simulink subsystem "brakePressure"  (R2023b)
settings: Solver=VariableStepAuto  StartTime=0.0  StopTime=10.0  RelTol=1e-3
libraries: brake_lib x4, Raptor_lib x4
settings Model: Creator=serga  LastModifiedBy=serga
settings OptimizationCC: ReuseModelBlockBuffer=off

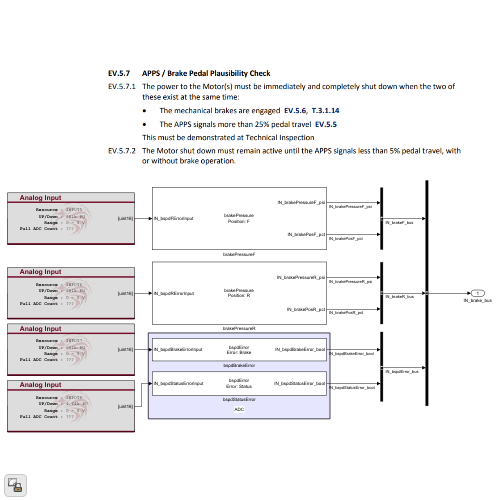
[thumbnail: Simulink's stored preview of the top-level diagram]
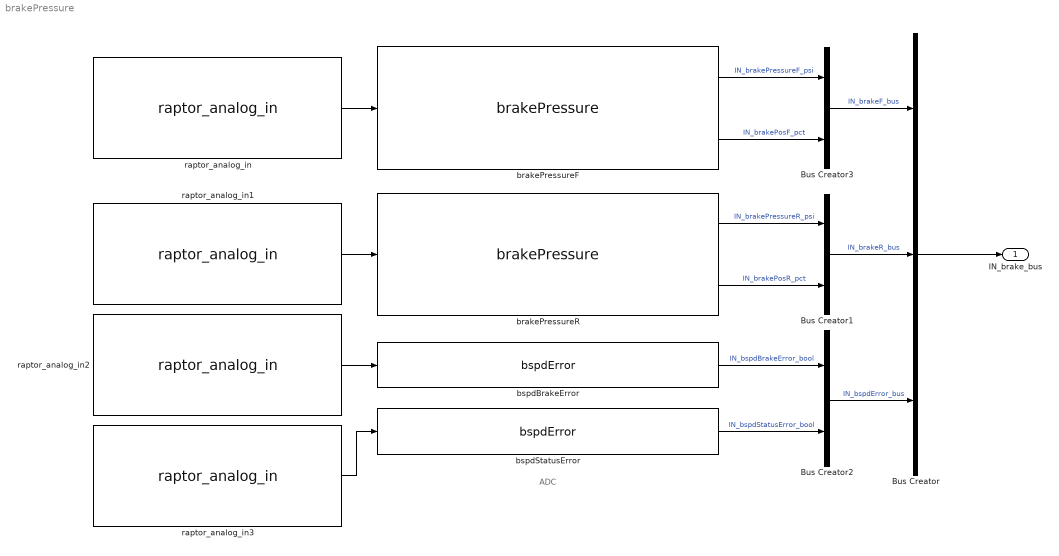
== system brakePressure ==
  note: ADC
  Bus Creator : BusCreator  Inputs=3
  Bus Creator1 : BusCreator  Inputs=2
  Bus Creator2 : BusCreator  Inputs=2
  Bus Creator3 : BusCreator  Inputs=2
  brakePressureF : brake_lib/brakePressure  pos='F'
  brakePressureR : brake_lib/brakePressure  pos='R'
  bspdBrakeError : brake_lib/bspdError  pos='Brake'
  bspdStatusError : brake_lib/bspdError  pos='Status'
  raptor_analog_in : Raptor_lib/Input & Output/raptor_analog_in  resourceValues=INPUT2|INPUT3|INPUT4|INPUT5|INPUT6|INPUT7|INPUT8|INPUT9|INPUT10|INPUT11|INPUT12|INPUT13|INPUT14|INPUT15|INPUT16|INPUT17|INPUT18|INPUT19|INPUT20|INPUT21|INPUT22|INPUT23|INPUT24|INPUT25|INPUT26|INPUT27|INPUT28|INPUT29|INPUT30|INPUT31|INPUT32|(None)  resource=INPUT4  rangeValues=0 - 5 V  range=0 - 5 V  filterrateValues=[]  filterrate='RAPTOR MASK DEFAULT'  resolutionValues=[]  resolution=[]  pullUDValues=422k PD  pullUD=422k PD
      settings: SourceProductName=Raptor
  raptor_analog_in1 : Raptor_lib/Input & Output/raptor_analog_in  resourceValues=INPUT2|INPUT3|INPUT4|INPUT5|INPUT6|INPUT7|INPUT8|INPUT9|INPUT10|INPUT11|INPUT12|INPUT13|INPUT14|INPUT15|INPUT16|INPUT17|INPUT18|INPUT19|INPUT20|INPUT21|INPUT22|INPUT23|INPUT24|INPUT25|INPUT26|INPUT27|INPUT28|INPUT29|INPUT30|INPUT31|INPUT32|(None)  resource=INPUT12  rangeValues=0 - 5 V  range=0 - 5 V  filterrateValues=[]  filterrate='RAPTOR MASK DEFAULT'  resolutionValues=[]  resolution=[]  pullUDValues=422k PD  pullUD=422k PD
      settings: SourceProductName=Raptor
  raptor_analog_in2 : Raptor_lib/Input & Output/raptor_analog_in  resourceValues=INPUT2|INPUT3|INPUT4|INPUT5|INPUT6|INPUT7|INPUT8|INPUT9|INPUT10|INPUT11|INPUT12|INPUT13|INPUT14|INPUT15|INPUT16|INPUT17|INPUT18|INPUT19|INPUT20|INPUT21|INPUT22|INPUT23|INPUT24|INPUT25|INPUT26|INPUT27|INPUT28|INPUT29|INPUT30|INPUT31|INPUT32|(None)  resource=INPUT17  rangeValues=0 - 5 V  range=0 - 5 V  filterrateValues=[]  filterrate='RAPTOR MASK DEFAULT'  resolutionValues=[]  resolution=[]  pullUDValues=422k PD  pullUD=422k PD
      settings: SourceProductName=Raptor
  raptor_analog_in3 : Raptor_lib/Input & Output/raptor_analog_in  resourceValues=INPUT2|INPUT3|INPUT4|INPUT5|INPUT6|INPUT7|INPUT8|INPUT9|INPUT10|INPUT11|INPUT12|INPUT13|INPUT14|INPUT15|INPUT16|INPUT17|INPUT18|INPUT19|INPUT20|INPUT21|INPUT22|INPUT23|INPUT24|INPUT25|INPUT26|INPUT27|INPUT28|INPUT29|INPUT30|INPUT31|INPUT32|(None)  resource=INPUT18  rangeValues=0 - 5 V  range=0 - 5 V  filterrateValues=[]  filterrate='RAPTOR MASK DEFAULT'  resolutionValues=[]  resolution=[]  pullUDValues=422k PD  pullUD=422k PD
      settings: SourceProductName=Raptor
  IN_brake_bus : Outport
  wires:
  Bus Creator2/1 -> Bus Creator/3  "IN_bspdError_bus"
  bspdStatusError/1 -> Bus Creator2/2  "IN_bspdStatusError_bool"
  bspdBrakeError/1 -> Bus Creator2/1  "IN_bspdBrakeError_bool"
  Bus Creator1/1 -> Bus Creator/2  "IN_brakeR_bus"
  Bus Creator3/1 -> Bus Creator/1  "IN_brakeF_bus"
  brakePressureR/2 -> Bus Creator1/2  "IN_brakePosR_pct"
  brakePressureR/1 -> Bus Creator1/1  "IN_brakePressureR_psi"
  brakePressureF/1 -> Bus Creator3/1  "IN_brakePressureF_psi"
  brakePressureF/2 -> Bus Creator3/2  "IN_brakePosF_pct"
  Bus Creator/1 -> IN_brake_bus/1
  raptor_analog_in/1 -> brakePressureF/1
  raptor_analog_in1/1 -> brakePressureR/1
  raptor_analog_in2/1 -> bspdBrakeError/1
  raptor_analog_in3/1 -> bspdStatusError/1
